simulink model "model_test_3_G_D_L_s_pro"  (R2015a)
settings: Solver=ode45  SolverMode=SingleTasking  StartTime=0.0  StopTime=100  RelTol=1e-6
values from neighbouring files (symbols this model uses):
  I_Dg = atan(((Xq*I_Pg - Ra*I_Qg)/I_Ug)/(I_Ug + (Ra*I_Pg + Xq*I_Qg)/I_Ug))    [Pal_GES.m]
  I_Dg_2 = atan(((Xq*I_Pd - Ra*I_Qg_2)/I_Ug)/(I_Ug + (Ra*I_Pd + Xq*I_Qg)/I_Ug))    [Pal_GES.m]
  I_ir = -I_id + I_Eiq/Xad    [Pal_GES.m]
  I_Mu = I_Mt    [Pal_GES.m]
  I_Mu_2 = I_Mt_2    [Pal_GES.m]
  I_ur = I_ir*Rr    [Pal_GES.m]
  I_Yd = Xd*I_id + Xad*I_ir    [Pal_GES.m]
  I_Yq = Xq*I_iq    [Pal_GES.m]
  I_Yr = I_Eiq + Xsf*I_ir    [Pal_GES.m]
  I_Yr_2 = I_Eiq_2 + Xsf*I_ir_2    [Pal_GES.m]
  I_Yrd = I_Eiq    [Pal_GES.m]
  I_Yrd_2 = I_Eiq_2    [Pal_GES.m]
  I_Yrq = -I_ud - I_iq*Xs - I_id*Ra    [Pal_GES.m]
  I_Yrq_2 = -I_ud - I_iq_2*Xs - I_id_2*Ra    [Pal_GES.m]
  N_Eq = N_ir*Xad    [Pal_GES.m]
  N_ur = N_ir*Rr    [Pal_GES.m]
  Ra = 3.236e-3    (= 0.003236)    [Pal_GES.m]
  Rl = 0.001    [Pal_GES.m]
  Rr = 8.75e-4    (= 0.000875)    [Pal_GES.m]
  Rrd = 8.75e-3    (= 0.00875)    [Pal_GES.m]
  Rrq = 8.75e-3    (= 0.00875)    [Pal_GES.m]
  Sigma = 0.0475    [Pal_GES.m]
  TauC = 0.8    [Pal_GES.m]
  Tj = 4    [Pal_GES.m]
  Wc = 100*pi    (= 314.159265359)    [Pal_GES.m]
  Xad = Xd - Xs    (= 0.6)    [Pal_GES.m]
  Xaq = Xq - Xs    (= 0.39)    [Pal_GES.m]
  Xd = 0.7    [Pal_GES.m]
  Xf = Xsf + Xad    (= 1)    [Pal_GES.m]
  Xl = 0.1    [Pal_GES.m]
  Xq = 0.49    [Pal_GES.m]
  Xrd = Xsrd + Xad    (= 0.936)    [Pal_GES.m]
  Xrq = Xsrq + Xaq    (= 0.6084)    [Pal_GES.m]
settings Model: Creator=art  LastModifiedBy=arti
settings SolverCC: ZeroCrossAlgorithm=Adaptive
settings DataIOCC: SignalLoggingSaveFormat=ModelDataLogs
settings OptimizationCC: BlockReduction=off  BooleanDataType=off  ExpressionDepthLimit=2147483647
settings DebuggingCC: SaveWithParameterizedLinksMsg=none  UnderspecifiedInitializationDetection=Classic  MergeDetectMultiDrivingBlocksExec=none  SignalResolutionControl=TryResolveAllWithWarning  MultiTaskDSMMsg=warning  MultiTaskCondExecSysMsg=none  StateNameClashWarn=warning
settings HardwareCC: TargetUnknown=on

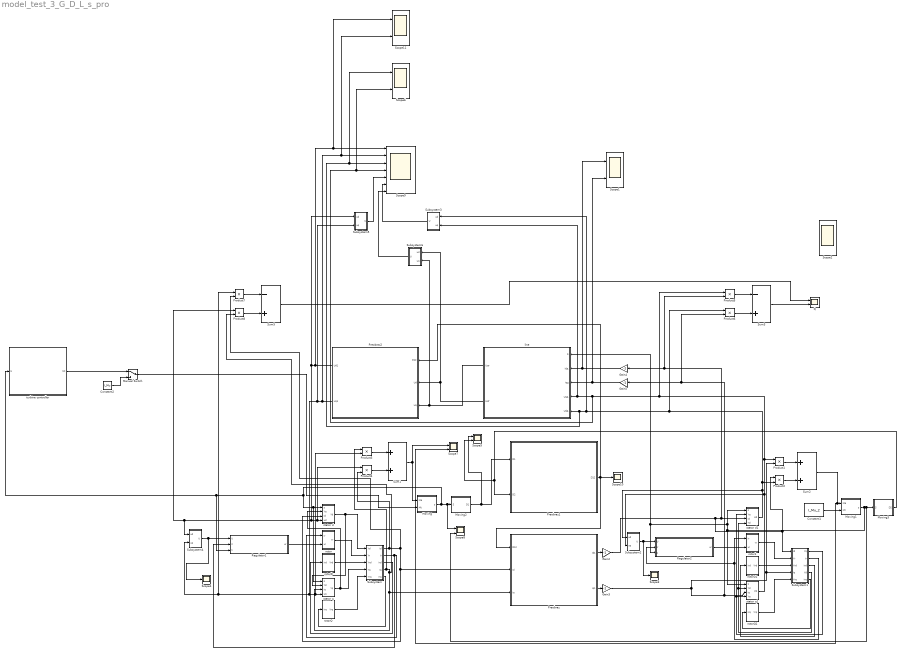
== system model_test_3_G_D_L_s_pro ==
  Constant1 : Constant  Value=I_Mu_2
  Constant2 : Constant  Value=I_Mu
  Gain{2..5} (4 alike) : Gain  Gain=-1
  Manual Switch : ManualSwitch
  Moving : Subsystem
  Moving1 : Subsystem
  Moving2 : Subsystem
  Moving3 : Subsystem
  Preobraz : Subsystem
  Preobraz1 : Subsystem
  Preobraz2 : Subsystem
  Product{1..8} (8 alike) : Product  RndMeth=Zero
  Q : Scope  NumInputPorts=2
      settings: YMin=-5~-5  YMax=5~5  SaveName=ScopeData4
  Regulator1 : Subsystem
  Regulator2 : Subsystem
  Scope{1,5..8,11} (6 alike) : Scope  NumInputPorts=2
      Scope1 settings: YMin=-5~-5  YMax=5~5  SaveName=ScopeData3
      Scope11 settings: TimeRange=21.65142549757934  YMin=-0.4124999999999991~0.875516528925619  YMax=-0.1647727272727264~1.006714876033057  SaveName=ScopeData15
      Scope5 settings: TimeRange=1.663515497972398  YMin=-4.39~-5  YMax=-4.22~5  SaveName=ScopeData9
      Scope6 settings: YMin=-5~-5  YMax=5~5  SaveName=ScopeData10
      Scope7 settings: TimeRange=1.663515497972398  YMin=-1~-5  YMax=1~5  SaveName=ScopeData11
      Scope8 settings: TimeRange=1.663515497972398  YMin=-0.380022~-5  YMax=-0.124479~5  SaveName=ScopeData12
  Scope10 : Scope
      settings: TimeRange=1.663515497972398  YMin=-0.380022  YMax=-0.124479  SaveName=ScopeData14
  Scope2 : Scope  NumInputPorts=6
      settings: YMin=-5~-5~-5~-5~-5~-5  YMax=5~5~5~5~5~5  SaveName=ScopeData6
  Scope3 : Scope
      settings: TimeRange=1.663515497972398  YMin=-0.3800219538968167  YMax=-0.1244785949506035  SaveName=ScopeData7
  Scope4 : Scope
      settings: TimeRange=1.663515497972398  YMin=-0.3800219538968167  YMax=-0.1244785949506035  SaveName=ScopeData8
  Scope9 : Scope  NumInputPorts=7
      settings: TimeRange=1.663515497972398  YMin=-0.380022~-5~-5~-5~-5~-5~-5  YMax=-0.124479~5~5~5~5~5~5  SaveName=ScopeData13
  Subsystem : Subsystem
  Subsystem1 : Subsystem
  Subsystem2 : Subsystem
  Subsystem3 : Subsystem
  Subsystem4 : Subsystem
  Subsystem5 : Subsystem
  Subsystem6 : Subsystem
  Sum1 : Sum
  Sum2 : Sum
  Sum3 : Sum  Inputs=-+
  Sum5 : Sum  Inputs=-+
  line : Subsystem
  rotor : Subsystem
  rotor1 : Subsystem
  rotorD : Subsystem
  rotorD1 : Subsystem
  rotorQ : Subsystem
  rotorQ1 : Subsystem
  stator d : Subsystem
  stator d1 : Subsystem
  stator q : Subsystem
  stator q1 : Subsystem
  turbine controller : Subsystem
  wires:
  rotor/1(Yr) -> Subsystem/2(Yr)
  rotorD/1(Yrd) -> Subsystem/3(Yrd)
  stator q/1(Yq) -> Subsystem/4(Yq), stator d/2(Yq)
  rotorQ/1(Yrq) -> Subsystem/5(Yrq)
  Subsystem/5(irq) -> rotorQ/1(irq)
  Subsystem/3(ird) -> rotorD/1(ird)
  Subsystem/2(ir) -> Regulator1/2(Ir), rotor/1(ir)
  stator d/1(Yd) -> stator q/2(Yd), Subsystem/1(Yd)
  Regulator1/1(ur) -> rotor/2(ur)
  rotor1/1(Yr) -> Subsystem1/2(Yr)
  rotorD1/1(Yrd) -> Subsystem1/3(Yrd)
  rotorQ1/1(Yrq) -> Subsystem1/5(Yrq)
  Subsystem1/5(irq) -> rotorQ1/1(irq)
  Subsystem1/4(Yd) -> stator q1/2(Yd), stator d1/4(Yd)
  Subsystem1/3(ird) -> rotorD1/1(ird)
  Subsystem1/2(ir) -> Regulator2/2(Ir), rotor1/1(ir)
  Regulator2/1(ur) -> rotor1/2(ur)
  Subsystem1/1(Yq) -> stator d1/2(Yq), stator q1/4(Yq)
  Constant1/1 -> Moving1/2(Mt)
  line/1(Uqг) -> Subsystem6/2(uq), Preobraz2/3(Uq)
  Preobraz1/1(D12) -> Preobraz/1(D12), Preobraz2/1(D12), Scope10/1
  Product3/1 -> Sum1/1
  Product4/1 -> Sum1/2
  Sum1/1 -> Scope7/1, Moving/1(Me)
  Product1/1 -> Sum2/1
  Product2/1 -> Sum2/2
  Moving2/1(D1) -> Scope5/1, Preobraz1/1(D1)
  Moving3/1(D2) -> Scope5/2, Preobraz1/2(D2)
  Subsystem2/1(U) -> Scope3/1, Regulator2/1(U)
  Subsystem4/1(U) -> Scope4/1, Regulator1/1(U)
  Moving/1(s) -> Scope8/1, Moving2/1(S), turbine controller/1(S), Regulator1/3(s), stator q/1(s), stator d/1(s)
  Moving1/1(s) -> Scope8/2, Moving3/1(S), Regulator2/3(s), line/1(S), stator d1/1(s), stator q1/1(s)
  Preobraz/1(Id1) -> Gain2/1
  Preobraz/2(Iq1) -> Gain3/1
  Sum2/1 -> Scope7/2, Moving1/1(Me)
  Gain2/1 -> Subsystem1/1(id), Product2/1, Product5/2, Gain4/1, stator d1/3(id)
  Gain3/1 -> Product6/2, Gain5/1, stator q1/3(iq), Subsystem1/4(iq), Product1/2
  stator d1/1(Ud) -> Subsystem2/1(ud), Product6/1, Subsystem3/1(ud), line/5(Udд), Scope6/1, Scope9/3, Product2/2
  stator q1/1(Uq) -> Subsystem2/2(uq), Product5/1, Subsystem3/2(uq), line/4(Uqд), Scope6/2, Scope9/4, Product1/1
  Gain4/1 -> Scope1/1, line/2(Idд)
  Gain5/1 -> Scope1/2, line/3(iqд)
  Subsystem5/1(U) -> Scope9/5
  Subsystem3/1(U) -> Scope9/6
  line/2(Udг) -> Preobraz2/2(Ud), Subsystem6/1(ud)
  Subsystem6/1(U) -> Scope9/7
  Product6/1 -> Sum3/2
  Product5/1 -> Sum3/1
  Sum3/1 -> Q/2
  Product8/1 -> Sum5/2
  Product7/1 -> Sum5/1
  Sum5/1 -> Q/1
  Preobraz2/2(Uq1) -> Subsystem5/2(uq), Product7/1, Subsystem4/2(uq), stator q/4(uq), Product3/2, Scope11/2, Scope9/2
  Subsystem/1(id) -> Product4/2, Product7/2, Preobraz/2(Id), stator d/3(id)
  Subsystem/4(iq) -> Product8/2, Preobraz/3(Iq), stator q/3(iq), Product3/1
  Preobraz2/1(Ud1) -> Product8/1, Subsystem4/1(ud), Product4/1, stator d/4(ud), Subsystem5/1(ud), Scope11/1, Scope9/1
  Manual Switch/1 -> Moving/2(Mt)
  Constant2/1 -> Manual Switch/2
  turbine controller/1(Mt) -> Manual Switch/1

== system model_test_3_G_D_L_s_pro/Moving ==
  Me : Inport
  Mt : Inport  Port=2
  Gain : Gain  Gain=1/Tj
  Integrator : Integrator
  Sum : Sum  Inputs=-+
  s : Outport
  wires:
  Sum/1 -> Gain/1
  Mt/1 -> Sum/2
  Me/1 -> Sum/1
  Gain/1 -> Integrator/1
  Integrator/1 -> s/1

== system model_test_3_G_D_L_s_pro/Moving1 ==
  Me : Inport
  Mt : Inport  Port=2
  Gain : Gain  Gain=1/Tj
  Integrator : Integrator
  Sum : Sum  Inputs=-+
  s : Outport
  wires:
  Sum/1 -> Gain/1
  Mt/1 -> Sum/2
  Me/1 -> Sum/1
  Gain/1 -> Integrator/1
  Integrator/1 -> s/1

== system model_test_3_G_D_L_s_pro/Moving2 ==
  S : Inport
  Gain1 : Gain  Gain=Wc
  Integrator1 : Integrator  InitialCondition=I_Dg
  D1 : Outport
  wires:
  Gain1/1 -> Integrator1/1
  Integrator1/1 -> D1/1
  S/1 -> Gain1/1

== system model_test_3_G_D_L_s_pro/Moving3 ==
  S : Inport
  Gain1 : Gain  Gain=Wc
  Integrator1 : Integrator  InitialCondition=I_Dg_2
  D2 : Outport
  wires:
  Gain1/1 -> Integrator1/1
  Integrator1/1 -> D2/1
  S/1 -> Gain1/1

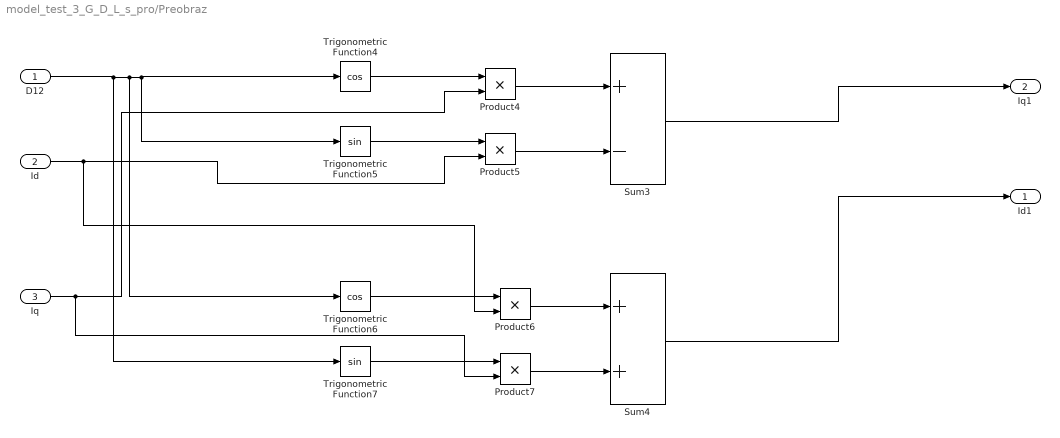
== system model_test_3_G_D_L_s_pro/Preobraz ==
  D12 : Inport
  Id : Inport  Port=2
  Iq : Inport  Port=3
  Product{4..7} (4 alike) : Product  RndMeth=Zero
  Sum3 : Sum  Inputs=+-
  Sum4 : Sum
  Trigonometric Function4 : Trigonometry  Operator=cos
  Trigonometric Function5 : Trigonometry
  Trigonometric Function6 : Trigonometry  Operator=cos
  Trigonometric Function7 : Trigonometry
  Id1 : Outport
  Iq1 : Outport  Port=2
  wires:
  Trigonometric Function4/1 -> Product4/1
  Trigonometric Function5/1 -> Product5/1
  Trigonometric Function6/1 -> Product6/1
  Trigonometric Function7/1 -> Product7/1
  D12/1 -> Trigonometric Function4/1, Trigonometric Function5/1, Trigonometric Function6/1, Trigonometric Function7/1
  Iq/1 -> Product7/2, Product4/2
  Id/1 -> Product6/2, Product5/2
  Product4/1 -> Sum3/1
  Product5/1 -> Sum3/2
  Product6/1 -> Sum4/1
  Product7/1 -> Sum4/2
  Sum4/1 -> Id1/1
  Sum3/1 -> Iq1/1

== system model_test_3_G_D_L_s_pro/Preobraz1 ==
  D1 : Inport
  D2 : Inport  Port=2
  Sum2 : Sum  Inputs=+-
  D12 : Outport
  wires:
  D2/1 -> Sum2/2
  D1/1 -> Sum2/1
  Sum2/1 -> D12/1

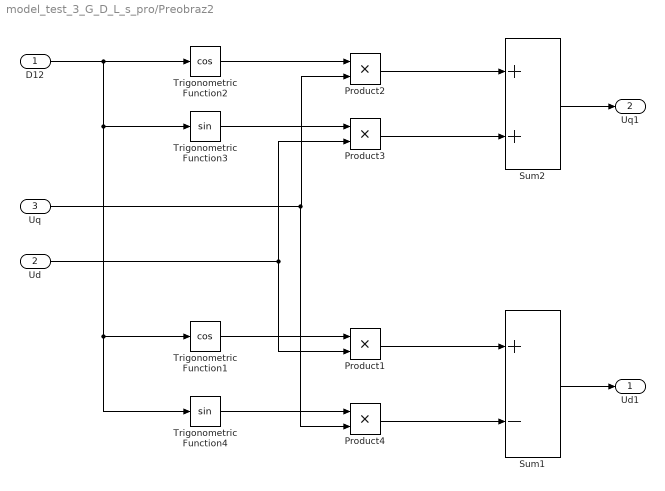
== system model_test_3_G_D_L_s_pro/Preobraz2 ==
  D12 : Inport
  Ud : Inport  Port=2
  Uq : Inport  Port=3
  Product{1..4} (4 alike) : Product  RndMeth=Zero
  Sum1 : Sum  Inputs=+-
  Sum2 : Sum
  Trigonometric Function1 : Trigonometry  Operator=cos
  Trigonometric Function2 : Trigonometry  Operator=cos
  Trigonometric Function3 : Trigonometry
  Trigonometric Function4 : Trigonometry
  Ud1 : Outport
  Uq1 : Outport  Port=2
  wires:
  Sum1/1 -> Ud1/1
  Sum2/1 -> Uq1/1
  Product4/1 -> Sum1/2
  Product1/1 -> Sum1/1
  Trigonometric Function4/1 -> Product4/1
  Trigonometric Function1/1 -> Product1/1
  Product3/1 -> Sum2/2
  Product2/1 -> Sum2/1
  Ud/1 -> Product3/2, Product1/2
  Uq/1 -> Product2/2, Product4/2
  Trigonometric Function3/1 -> Product3/1
  Trigonometric Function2/1 -> Product2/1
  D12/1 -> Trigonometric Function4/1, Trigonometric Function1/1, Trigonometric Function3/1, Trigonometric Function2/1

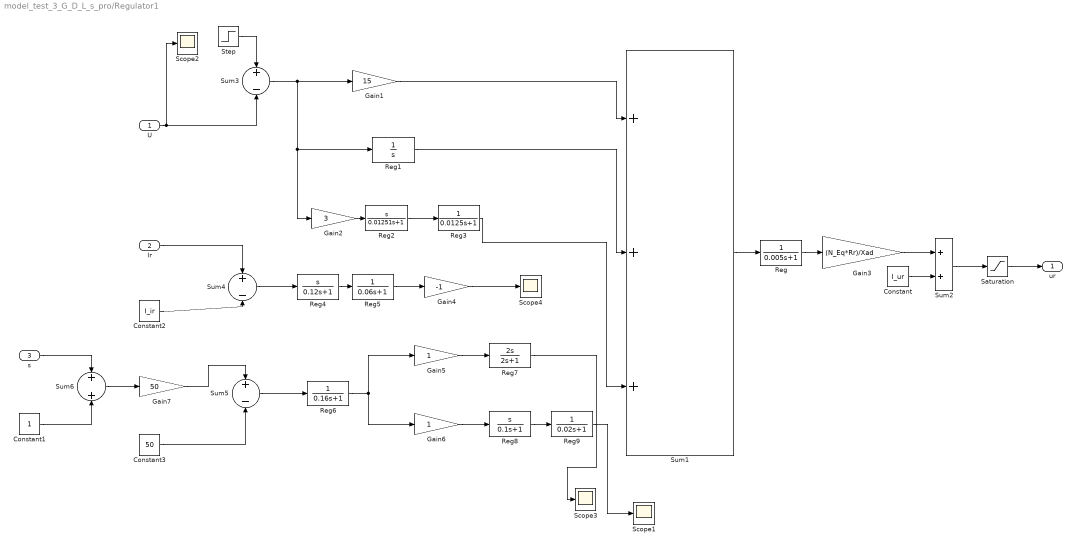
== system model_test_3_G_D_L_s_pro/Regulator1 ==
  U : Inport
  Ir : Inport  Port=2
  s : Inport  Port=3
  Constant : Constant  Value=I_ur
  Constant1 : Constant
  Constant2 : Constant  Value=I_ir
  Constant3 : Constant  Value=50
  Gain1 : Gain  Gain=15
  Gain2 : Gain  Gain=3
  Gain3 : Gain  Gain=(N_Eq*Rr)/Xad
  Gain4 : Gain  Gain=-1
  Gain5 : Gain
  Gain6 : Gain
  Gain7 : Gain  Gain=50
  Reg : TransferFcn  Numerator=1  Denominator=[0.005 1]
  Reg1 : TransferFcn  Numerator=1  Denominator=[1 0]
  Reg2 : TransferFcn  Numerator=[1 0]  Denominator=[0.01251 1]
  Reg3 : TransferFcn  Numerator=1  Denominator=[0.0125 1]
  Reg4 : TransferFcn  Numerator=[1 0]  Denominator=[0.12 1]
  Reg5 : TransferFcn  Numerator=1  Denominator=[0.06 1]
  Reg6 : TransferFcn  Numerator=[1 ]  Denominator=[0.16 1]
  Reg7 : TransferFcn  Numerator=[2 0]  Denominator=[2 1]
  Reg8 : TransferFcn  Numerator=[1 0]  Denominator=[0.1 1]
  Reg9 : TransferFcn  Denominator=[0.02 1]
  Saturation : Saturate  UpperLimit=2*N_ur  LowerLimit=-N_ur
  Scope{1..4} (4 alike) : Scope
      Scope1 settings: TimeRange=3.056721056721056  YMin=0.4  YMax=0.65
      Scope2 settings: TimeRange=3.056721056721056  YMin=0.4  YMax=0.65  SaveName=ScopeData5
      Scope3 settings: TimeRange=3.056721056721056  YMin=0.4  YMax=0.65  SaveName=ScopeData2
      Scope4 settings: TimeRange=3.056721056721056  YMin=0.4  YMax=0.65
  Step : Step  Time=50  Before=1  After=1.0  SampleTime=0
  Sum1 : Sum  Inputs=+++
  Sum2 : Sum
  Sum3 : Sum  Inputs=+-
  Sum4 : Sum  Inputs=+-
  Sum5 : Sum  Inputs=+-
  Sum6 : Sum
  ur : Outport
  wires:
  Gain3/1 -> Sum2/1
  Constant/1 -> Sum2/2
  U/1 -> Sum3/2, Scope2/1
  Reg/1 -> Gain3/1
  Sum2/1 -> Saturation/1
  Saturation/1 -> ur/1
  Reg1/1 -> Sum1/2
  Gain1/1 -> Sum1/1
  Sum1/1 -> Reg/1
  Gain2/1 -> Reg2/1
  Reg2/1 -> Reg3/1
  Reg3/1 -> Sum1/3
  Sum3/1 -> Gain2/1, Reg1/1, Gain1/1
  Reg5/1 -> Gain4/1
  Ir/1 -> Sum4/1
  Constant2/1 -> Sum4/2
  Sum4/1 -> Reg4/1
  Reg4/1 -> Reg5/1
  Constant1/1 -> Sum6/2
  Gain5/1 -> Reg7/1
  Reg6/1 -> Gain5/1, Gain6/1
  Gain6/1 -> Reg8/1
  Reg8/1 -> Reg9/1
  s/1 -> Sum6/1
  Sum6/1 -> Gain7/1
  Gain7/1 -> Sum5/1
  Sum5/1 -> Reg6/1
  Constant3/1 -> Sum5/2
  Reg9/1 -> Scope1/1
  Reg7/1 -> Scope3/1
  Step/1 -> Sum3/1
  Gain4/1 -> Scope4/1

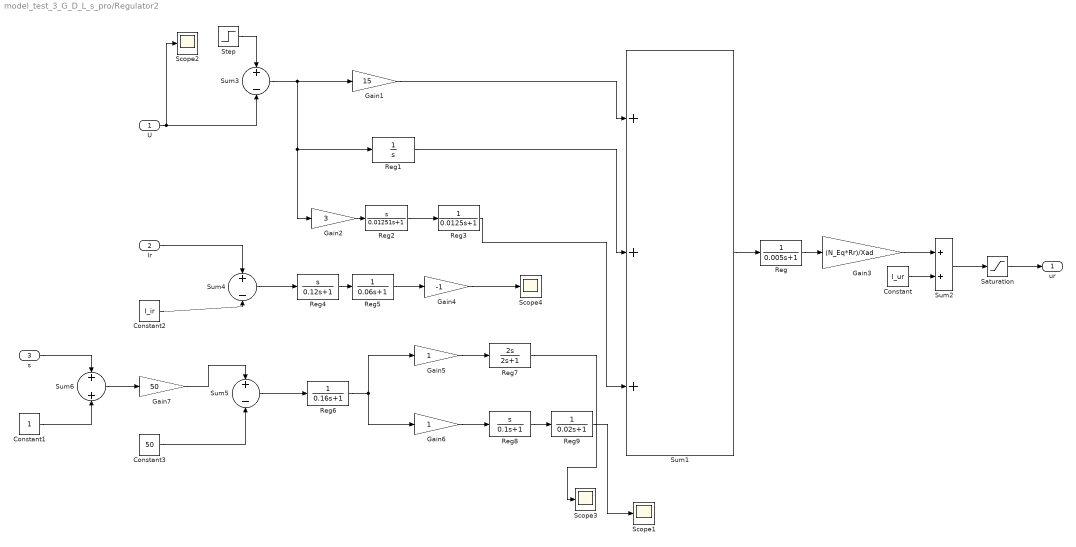
== system model_test_3_G_D_L_s_pro/Regulator2 ==
  U : Inport
  Ir : Inport  Port=2
  s : Inport  Port=3
  Constant : Constant  Value=I_ur
  Constant1 : Constant
  Constant2 : Constant  Value=I_ir
  Constant3 : Constant  Value=50
  Gain1 : Gain  Gain=15
  Gain2 : Gain  Gain=3
  Gain3 : Gain  Gain=(N_Eq*Rr)/Xad
  Gain4 : Gain  Gain=-1
  Gain5 : Gain
  Gain6 : Gain
  Gain7 : Gain  Gain=50
  Reg : TransferFcn  Numerator=1  Denominator=[0.005 1]
  Reg1 : TransferFcn  Numerator=1  Denominator=[1 0]
  Reg2 : TransferFcn  Numerator=[1 0]  Denominator=[0.01251 1]
  Reg3 : TransferFcn  Numerator=1  Denominator=[0.0125 1]
  Reg4 : TransferFcn  Numerator=[1 0]  Denominator=[0.12 1]
  Reg5 : TransferFcn  Numerator=1  Denominator=[0.06 1]
  Reg6 : TransferFcn  Numerator=[1 ]  Denominator=[0.16 1]
  Reg7 : TransferFcn  Numerator=[2 0]  Denominator=[2 1]
  Reg8 : TransferFcn  Numerator=[1 0]  Denominator=[0.1 1]
  Reg9 : TransferFcn  Denominator=[0.02 1]
  Saturation : Saturate  UpperLimit=2*N_ur  LowerLimit=-N_ur
  Scope{1..4} (4 alike) : Scope
      Scope1 settings: TimeRange=3.056721056721056  YMin=0.4  YMax=0.65
      Scope2 settings: TimeRange=3.056721056721056  YMin=0.4  YMax=0.65  SaveName=ScopeData5
      Scope3 settings: TimeRange=3.056721056721056  YMin=0.4  YMax=0.65  SaveName=ScopeData2
      Scope4 settings: TimeRange=3.056721056721056  YMin=0.4  YMax=0.65
  Step : Step  Time=0  Before=1  After=1.0  SampleTime=0
  Sum1 : Sum  Inputs=+++
  Sum2 : Sum
  Sum3 : Sum  Inputs=+-
  Sum4 : Sum  Inputs=+-
  Sum5 : Sum  Inputs=+-
  Sum6 : Sum
  ur : Outport
  wires:
  Gain3/1 -> Sum2/1
  Constant/1 -> Sum2/2
  U/1 -> Sum3/2, Scope2/1
  Reg/1 -> Gain3/1
  Sum2/1 -> Saturation/1
  Saturation/1 -> ur/1
  Reg1/1 -> Sum1/2
  Gain1/1 -> Sum1/1
  Sum1/1 -> Reg/1
  Gain2/1 -> Reg2/1
  Reg2/1 -> Reg3/1
  Reg3/1 -> Sum1/3
  Sum3/1 -> Gain2/1, Reg1/1, Gain1/1
  Reg5/1 -> Gain4/1
  Ir/1 -> Sum4/1
  Constant2/1 -> Sum4/2
  Sum4/1 -> Reg4/1
  Reg4/1 -> Reg5/1
  Constant1/1 -> Sum6/2
  Gain5/1 -> Reg7/1
  Reg6/1 -> Gain5/1, Gain6/1
  Gain6/1 -> Reg8/1
  Reg8/1 -> Reg9/1
  s/1 -> Sum6/1
  Sum6/1 -> Gain7/1
  Gain7/1 -> Sum5/1
  Sum5/1 -> Reg6/1
  Constant3/1 -> Sum5/2
  Reg9/1 -> Scope1/1
  Reg7/1 -> Scope3/1
  Step/1 -> Sum3/1
  Gain4/1 -> Scope4/1

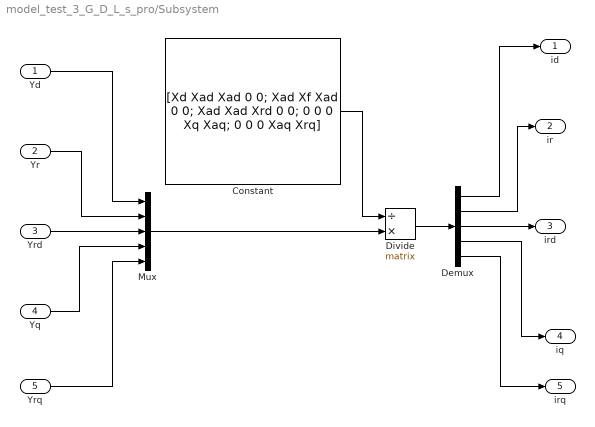
== system model_test_3_G_D_L_s_pro/Subsystem ==
  Yd : Inport
  Yr : Inport  Port=2
  Yrd : Inport  Port=3
  Yq : Inport  Port=4
  Yrq : Inport  Port=5
  Constant : Constant  Value=[Xd Xad Xad 0 0; Xad Xf Xad 0 0; Xad Xad Xrd 0 0; 0 0 0 Xq Xaq; 0 0 0 Xaq Xrq]  VectorParams1D=off
  Demux : Demux  Outputs=5
  Divide : Product  Inputs=/*  Multiplication=Matrix(*)
  Mux : Mux  Inputs=5
  id : Outport
  ir : Outport  Port=2
  ird : Outport  Port=3
  iq : Outport  Port=4
  irq : Outport  Port=5
  wires:
  Mux/1 -> Divide/2
  Yrd/1 -> Mux/3
  Yq/1 -> Mux/4
  Yrq/1 -> Mux/5
  Yr/1 -> Mux/2
  Yd/1 -> Mux/1
  Divide/1 -> Demux/1
  Demux/3 -> ird/1
  Demux/5 -> irq/1
  Demux/2 -> ir/1
  Demux/1 -> id/1
  Constant/1 -> Divide/1
  Demux/4 -> iq/1

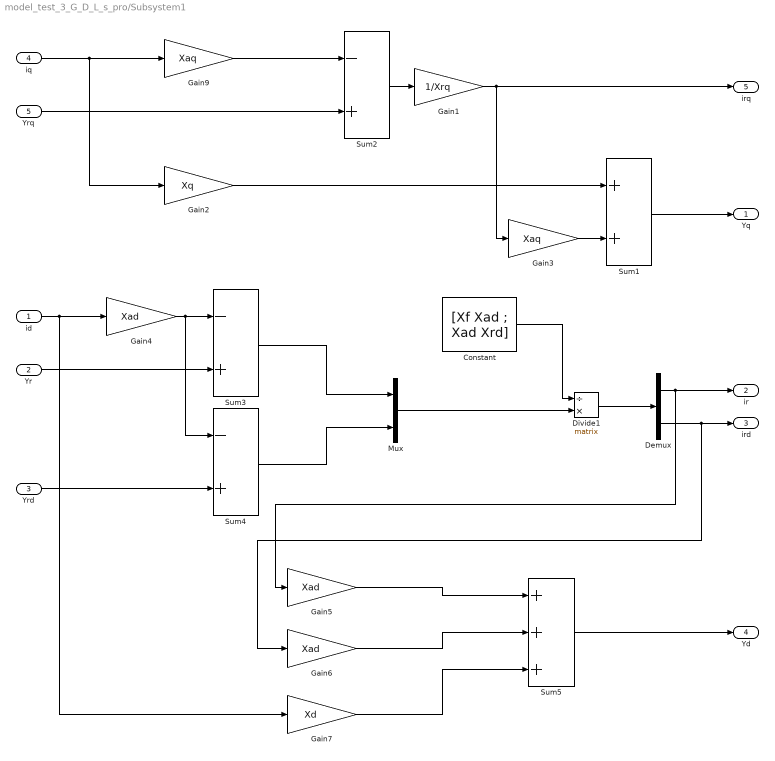
== system model_test_3_G_D_L_s_pro/Subsystem1 ==
  id : Inport
  Yr : Inport  Port=2
  Yrd : Inport  Port=3
  iq : Inport  Port=4
  Yrq : Inport  Port=5
  Constant : Constant  Value=[Xf Xad ; Xad Xrd]  VectorParams1D=off
  Demux : Demux  Outputs=2
  Divide1 : Product  Inputs=/*  Multiplication=Matrix(*)
  Gain1 : Gain  Gain=1/Xrq
  Gain2 : Gain  Gain=Xq
  Gain3 : Gain  Gain=Xaq
  Gain4 : Gain  Gain=Xad
  Gain5 : Gain  Gain=Xad
  Gain6 : Gain  Gain=Xad
  Gain7 : Gain  Gain=Xd
  Gain9 : Gain  Gain=Xaq
  Mux : Mux  Inputs=2
  Sum1 : Sum
  Sum2 : Sum  Inputs=-+
  Sum3 : Sum  Inputs=-+
  Sum4 : Sum  Inputs=-+
  Sum5 : Sum  Inputs=+++
  Yq : Outport
  ir : Outport  Port=2
  ird : Outport  Port=3
  Yd : Outport  Port=4
  irq : Outport  Port=5
  wires:
  Mux/1 -> Divide1/2
  Divide1/1 -> Demux/1
  iq/1 -> Gain2/1, Gain9/1
  Yrq/1 -> Sum2/2
  Gain9/1 -> Sum2/1
  Sum2/1 -> Gain1/1
  Gain1/1 -> Gain3/1, irq/1
  Gain2/1 -> Sum1/1
  Gain3/1 -> Sum1/2
  Sum1/1 -> Yq/1
  id/1 -> Gain7/1, Gain4/1
  Gain4/1 -> Sum4/1, Sum3/1
  Yr/1 -> Sum3/2
  Sum3/1 -> Mux/1
  Yrd/1 -> Sum4/2
  Sum4/1 -> Mux/2
  Constant/1 -> Divide1/1
  Demux/1 -> Gain5/1, ir/1
  Sum5/1 -> Yd/1
  Demux/2 -> Gain6/1, ird/1
  Gain5/1 -> Sum5/1
  Gain6/1 -> Sum5/2
  Gain7/1 -> Sum5/3

== system model_test_3_G_D_L_s_pro/Subsystem2 ==
  ud : Inport
  uq : Inport  Port=2
  Math Function : Math  Operator=square  SaturateOnIntegerOverflow=on
  Math Function1 : Math  Operator=square  SaturateOnIntegerOverflow=on
  Sqrt : Sqrt  SaturateOnIntegerOverflow=on
  Sum1 : Sum
  U : Outport
  wires:
  ud/1 -> Math Function/1
  uq/1 -> Math Function1/1
  Math Function1/1 -> Sum1/1
  Math Function/1 -> Sum1/2
  Sum1/1 -> Sqrt/1
  Sqrt/1 -> U/1

== system model_test_3_G_D_L_s_pro/Subsystem3 ==
  ud : Inport
  uq : Inport  Port=2
  Math Function : Math  Operator=square  SaturateOnIntegerOverflow=on
  Math Function1 : Math  Operator=square  SaturateOnIntegerOverflow=on
  Sqrt : Sqrt  SaturateOnIntegerOverflow=on
  Sum1 : Sum
  U : Outport
  wires:
  ud/1 -> Math Function/1
  uq/1 -> Math Function1/1
  Math Function1/1 -> Sum1/1
  Math Function/1 -> Sum1/2
  Sum1/1 -> Sqrt/1
  Sqrt/1 -> U/1

== system model_test_3_G_D_L_s_pro/Subsystem4 ==
  ud : Inport
  uq : Inport  Port=2
  Math Function : Math  Operator=square  SaturateOnIntegerOverflow=on
  Math Function1 : Math  Operator=square  SaturateOnIntegerOverflow=on
  Sqrt : Sqrt  SaturateOnIntegerOverflow=on
  Sum1 : Sum
  U : Outport
  wires:
  ud/1 -> Math Function/1
  uq/1 -> Math Function1/1
  Math Function1/1 -> Sum1/1
  Math Function/1 -> Sum1/2
  Sum1/1 -> Sqrt/1
  Sqrt/1 -> U/1

== system model_test_3_G_D_L_s_pro/Subsystem5 ==
  ud : Inport
  uq : Inport  Port=2
  Math Function : Math  Operator=square  SaturateOnIntegerOverflow=on
  Math Function1 : Math  Operator=square  SaturateOnIntegerOverflow=on
  Sqrt : Sqrt  SaturateOnIntegerOverflow=on
  Sum1 : Sum
  U : Outport
  wires:
  ud/1 -> Math Function/1
  uq/1 -> Math Function1/1
  Math Function1/1 -> Sum1/1
  Math Function/1 -> Sum1/2
  Sum1/1 -> Sqrt/1
  Sqrt/1 -> U/1

== system model_test_3_G_D_L_s_pro/Subsystem6 ==
  ud : Inport
  uq : Inport  Port=2
  Math Function : Math  Operator=square  SaturateOnIntegerOverflow=on
  Math Function1 : Math  Operator=square  SaturateOnIntegerOverflow=on
  Sqrt : Sqrt  SaturateOnIntegerOverflow=on
  Sum1 : Sum
  U : Outport
  wires:
  ud/1 -> Math Function/1
  uq/1 -> Math Function1/1
  Math Function1/1 -> Sum1/1
  Math Function/1 -> Sum1/2
  Sum1/1 -> Sqrt/1
  Sqrt/1 -> U/1

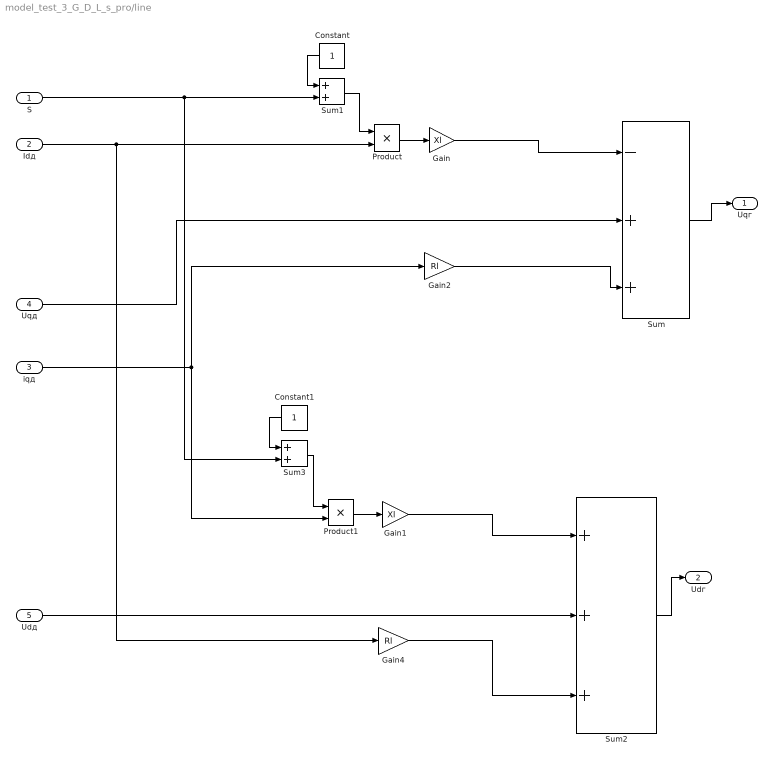
== system model_test_3_G_D_L_s_pro/line ==
  S : Inport
  Idд : Inport  Port=2
  iqд : Inport  Port=3
  Uqд : Inport  Port=4
  Udд : Inport  Port=5
  Constant : Constant
  Constant1 : Constant
  Gain : Gain  Gain=Xl
  Gain1 : Gain  Gain=Xl
  Gain2 : Gain  Gain=Rl
  Gain4 : Gain  Gain=Rl
  Product : Product  RndMeth=Zero
  Product1 : Product  RndMeth=Zero
  Sum : Sum  Inputs=-++
  Sum1 : Sum
  Sum2 : Sum  Inputs=+++
  Sum3 : Sum
  Uqг : Outport
  Udг : Outport  Port=2
  wires:
  Sum/1 -> Uqг/1
  Sum1/1 -> Product/1
  Constant/1 -> Sum1/1
  Product/1 -> Gain/1
  Gain/1 -> Sum/1
  Gain2/1 -> Sum/3
  Uqд/1 -> Sum/2
  Sum2/1 -> Udг/1
  S/1 -> Sum3/2, Sum1/2
  Sum3/1 -> Product1/1
  Constant1/1 -> Sum3/1
  Product1/1 -> Gain1/1
  Gain1/1 -> Sum2/1
  Gain4/1 -> Sum2/3
  iqд/1 -> Product1/2, Gain2/1
  Udд/1 -> Sum2/2
  Idд/1 -> Gain4/1, Product/2

== system model_test_3_G_D_L_s_pro/rotor ==
  ir : Inport
  ur : Inport  Port=2
  Gain : Gain  Gain=Wc
  Gain1 : Gain  Gain=Rr
  I1 : Integrator  InitialCondition=I_Yr
  Sum : Sum  Inputs=-+
  Yr : Outport
  wires:
  Sum/1 -> Gain/1
  I1/1 -> Yr/1
  Gain/1 -> I1/1
  ir/1 -> Gain1/1
  Gain1/1 -> Sum/1
  ur/1 -> Sum/2

== system model_test_3_G_D_L_s_pro/rotor1 ==
  ir : Inport
  ur : Inport  Port=2
  Gain : Gain  Gain=Wc
  Gain1 : Gain  Gain=Rr
  I1 : Integrator  InitialCondition=I_Yr_2
  Sum : Sum  Inputs=-+
  Yr : Outport
  wires:
  Sum/1 -> Gain/1
  I1/1 -> Yr/1
  Gain/1 -> I1/1
  ir/1 -> Gain1/1
  Gain1/1 -> Sum/1
  ur/1 -> Sum/2

== system model_test_3_G_D_L_s_pro/rotorD ==
  ird : Inport
  Gain : Gain  Gain=Wc
  Gain1 : Gain  Gain=Rrd
  Gain2 : Gain  Gain=-1
  I1 : Integrator  InitialCondition=I_Yrd
  Yrd : Outport
  wires:
  Gain1/1 -> Gain/1
  I1/1 -> Yrd/1
  Gain/1 -> I1/1
  Gain2/1 -> Gain1/1
  ird/1 -> Gain2/1

== system model_test_3_G_D_L_s_pro/rotorD1 ==
  ird : Inport
  Gain : Gain  Gain=Wc
  Gain1 : Gain  Gain=Rrd
  Gain2 : Gain  Gain=-1
  I1 : Integrator  InitialCondition=I_Yrd_2
  Yrd : Outport
  wires:
  Gain1/1 -> Gain/1
  I1/1 -> Yrd/1
  Gain/1 -> I1/1
  Gain2/1 -> Gain1/1
  ird/1 -> Gain2/1

== system model_test_3_G_D_L_s_pro/rotorQ ==
  irq : Inport
  Gain : Gain  Gain=Wc
  Gain1 : Gain  Gain=Rrq
  Gain2 : Gain  Gain=-1
  I1 : Integrator  InitialCondition=I_Yrq
  Yrq : Outport
  wires:
  Gain1/1 -> Gain/1
  I1/1 -> Yrq/1
  Gain/1 -> I1/1
  Gain2/1 -> Gain1/1
  irq/1 -> Gain2/1

== system model_test_3_G_D_L_s_pro/rotorQ1 ==
  irq : Inport
  Gain : Gain  Gain=Wc
  Gain1 : Gain  Gain=Rrq
  Gain2 : Gain  Gain=-1
  I1 : Integrator  InitialCondition=I_Yrq_2
  Yrq : Outport
  wires:
  Gain1/1 -> Gain/1
  I1/1 -> Yrq/1
  Gain/1 -> I1/1
  Gain2/1 -> Gain1/1
  irq/1 -> Gain2/1

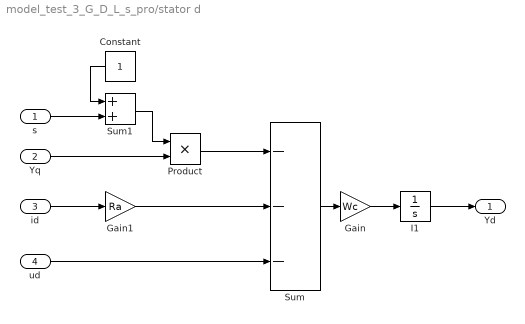
== system model_test_3_G_D_L_s_pro/stator d ==
  s : Inport
  Yq : Inport  Port=2
  id : Inport  Port=3
  ud : Inport  Port=4
  Constant : Constant
  Gain : Gain  Gain=Wc
  Gain1 : Gain  Gain=Ra
  I1 : Integrator  InitialCondition=I_Yd
  Product : Product  RndMeth=Zero
  Sum : Sum  Inputs=---
  Sum1 : Sum
  Yd : Outport
  wires:
  Sum/1 -> Gain/1
  I1/1 -> Yd/1
  ud/1 -> Sum/3
  Gain/1 -> I1/1
  id/1 -> Gain1/1
  s/1 -> Sum1/2
  Gain1/1 -> Sum/2
  Yq/1 -> Product/2
  Sum1/1 -> Product/1
  Product/1 -> Sum/1
  Constant/1 -> Sum1/1

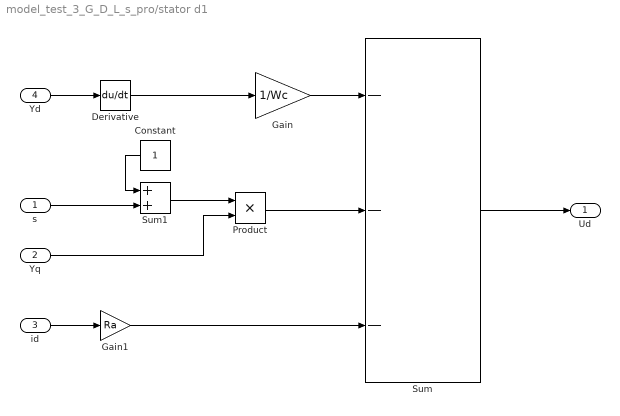
== system model_test_3_G_D_L_s_pro/stator d1 ==
  s : Inport
  Yq : Inport  Port=2
  id : Inport  Port=3
  Yd : Inport  Port=4
  Constant : Constant
  Derivative : Derivative  CoefficientInTFapproximation=I_Yd_2
  Gain : Gain  Gain=1/Wc
  Gain1 : Gain  Gain=Ra
  Product : Product  RndMeth=Zero
  Sum : Sum  Inputs=---
  Sum1 : Sum
  Ud : Outport
  wires:
  Gain/1 -> Sum/1
  Yd/1 -> Derivative/1
  Sum1/1 -> Product/1
  Constant/1 -> Sum1/1
  s/1 -> Sum1/2
  Yq/1 -> Product/2
  id/1 -> Gain1/1
  Product/1 -> Sum/2
  Gain1/1 -> Sum/3
  Sum/1 -> Ud/1
  Derivative/1 -> Gain/1

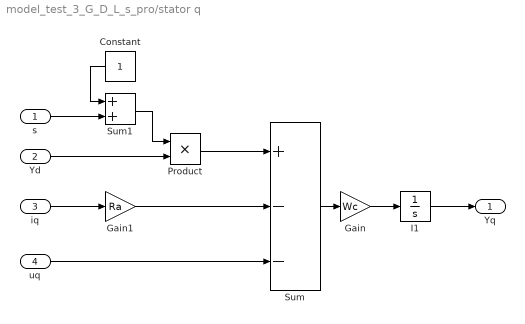
== system model_test_3_G_D_L_s_pro/stator q ==
  s : Inport
  Yd : Inport  Port=2
  iq : Inport  Port=3
  uq : Inport  Port=4
  Constant : Constant
  Gain : Gain  Gain=Wc
  Gain1 : Gain  Gain=Ra
  I1 : Integrator  InitialCondition=I_Yq
  Product : Product  RndMeth=Zero
  Sum : Sum  Inputs=+--
  Sum1 : Sum
  Yq : Outport
  wires:
  Sum/1 -> Gain/1
  I1/1 -> Yq/1
  uq/1 -> Sum/3
  Gain/1 -> I1/1
  iq/1 -> Gain1/1
  s/1 -> Sum1/2
  Gain1/1 -> Sum/2
  Yd/1 -> Product/2
  Sum1/1 -> Product/1
  Product/1 -> Sum/1
  Constant/1 -> Sum1/1

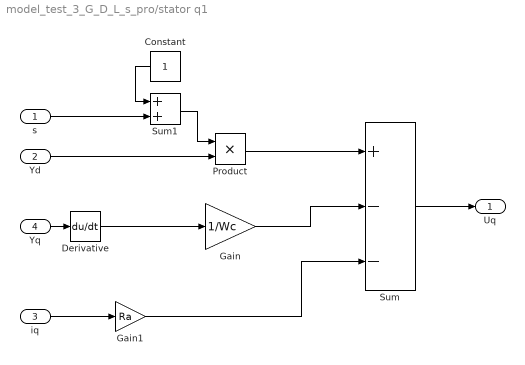
== system model_test_3_G_D_L_s_pro/stator q1 ==
  s : Inport
  Yd : Inport  Port=2
  iq : Inport  Port=3
  Yq : Inport  Port=4
  Constant : Constant
  Derivative : Derivative  CoefficientInTFapproximation=I_Yq_2
  Gain : Gain  Gain=1/Wc
  Gain1 : Gain  Gain=Ra
  Product : Product  RndMeth=Zero
  Sum : Sum  Inputs=+--
  Sum1 : Sum
  Uq : Outport
  wires:
  Sum1/1 -> Product/1
  Product/1 -> Sum/1
  Constant/1 -> Sum1/1
  s/1 -> Sum1/2
  Yd/1 -> Product/2
  Yq/1 -> Derivative/1
  iq/1 -> Gain1/1
  Gain/1 -> Sum/2
  Gain1/1 -> Sum/3
  Sum/1 -> Uq/1
  Derivative/1 -> Gain/1

== system model_test_3_G_D_L_s_pro/turbine controller ==
  S : Inport
  Constant4 : Constant  Value=I_Mu
  Gain : Gain  Gain=1/TauC
  Gain1 : Gain  Gain=1/Sigma
  Integrator : Integrator
  Sum4 : Sum  Inputs=-+-
  Mt : Outport
  wires:
  S/1 -> Gain1/1
  Gain/1 -> Integrator/1
  Constant4/1 -> Sum4/2
  Gain1/1 -> Sum4/1
  Integrator/1 -> Mt/1, Sum4/3
  Sum4/1 -> Gain/1
